simulink model "test4"  (Simulink 2.20)
settings: Solver=ode45  StartTime=0.0  StopTime=10.0  RelTol=1e-3  AbsTol=1e-6
settings Model: ConsistencyChecking=off  RTWPlaceOutputsASAP=off

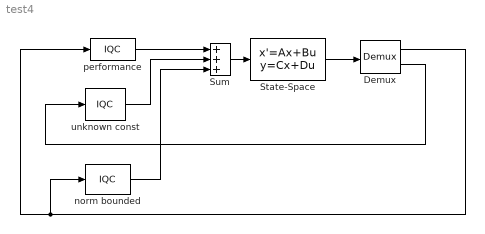
== system test4 ==
  Demux : Demux  Outputs=2
  State-Space : StateSpace  A=[-5,1;2,-3]  B=[0;1]  C=eye(2)  D=[0;0]  X0=0
  Sum : Sum  Inputs=+++
  norm bounded : S-Function  FunctionName=IQC  PortCounts=[]  SFunctionModules=''  mask(IQC block){@1=1, @2=v==iqc_ltvnorm(v);}
      mask prompts: @1 "Order"; @2 "List of iqc relationships:"
      mask help: Uncertain blocks specification
      mask Help: IQC block to contain any type of uncertainty
      mask Display: plot(0,0,100,100,[7,7],[20,80],[13,13],[20,80],[32,47,17,32],[70,35,35,70],[53,53],[20,80],[59,59],[20,80],[76,64,76],[38,50,63],[86,86,86,85,84,82],[29,54,59,62,65,67],[98,95,92,90,89,87,86],[66,67,66,62,59,55,52])
  performance : S-Function  FunctionName=IQC  PortCounts=[]  SFunctionModules=''  mask(IQC block){@1=1, @2=IN=w;OUT=f;}
      mask prompts: @1 "Order"; @2 "List of iqc relationships:"
      mask help: Uncertain blocks specification
      mask Help: IQC block to contain any type of uncertainty
      mask Display: plot(0,0,100,100,[10,20,30,40,30,20,10,0],[50,20,20,50,80,80,50,50],[90,80,70,60,70,80,90,100],[50,20,20,50,80,80,50,50],[55,45],[75,75],[55,45],[65,65],[55,45],[55,55],[46,55],[46,46],[55,46],[35,35],[55,46],[25,25])
  unknown const : S-Function  FunctionName=IQC  PortCounts=[]  SFunctionModules=''  mask(IQC block){@1=1, @2=v==iqc_ltigain(w);}
      mask prompts: @1 "Order"; @2 "List of iqc relationships:"
      mask help: Uncertain blocks specification
      mask Help: IQC block to contain any type of uncertainty
      mask Display: plot(0,0,100,100,[18,18],[27,72],[40,40,39,36,30,27,26,26,28,31,36,39],[68,31,30,29,29,32,37,42,46,49,49,48],[49,49],[27,73],[66,54,66],[40,50,58],[75,78],[63,67],[78,78],[30,67],[83,73],[30,30],[10,90,90,10,10],[88,88,12,12,88],[1,10],[50,50],[100,90],[50,50])
  wires:
  Demux/1 -> performance/1, norm bounded/1
  State-Space/1 -> Demux/1
  Demux/2 -> unknown const/1
  norm bounded/1 -> Sum/3
  performance/1 -> Sum/1
  unknown const/1 -> Sum/2
  Sum/1 -> State-Space/1
